simulink model "Sat_Nonliner_3"  (R2024a)
settings: Solver=ode45  StartTime=0.0  StopTime=20000  RelTol=1e-3  EnableMultiTasking=on
model workspace (MAT data in the model file):
  Q_fenzi = [2.841 -4.406 1.749]
values from neighbouring files (symbols this model uses):
  kzq_fenmu = kzq_fenmu_3    [Sat_Model_N_P.m]
  kzq_fenzi = kzq_fenzi_3    [Sat_Model_N_P.m]
  N_fenmu = N_fenmu_3    [Sat_Model_N_P.m]
  N_fenzi = N_fenzi_3    [Sat_Model_N_P.m]
  sat_alpha = sat_alpha_set_3_main(sat_alpha_i)    [SAT_MAIN.m]    (also in Sat_Model_G.m = 5; Sat_Model_N_P.m = sat_alpha_set(sat_alpha_i); model_sat_n_p.m = sat_alpha_1)
  T_fenmu = T_fenmu_3    [Sat_Model_N_P.m]
  T_fenzi = T_fenzi_3    [Sat_Model_N_P.m]
settings Model: Creator=75499  LastModifiedBy=xthinking
settings SolverCC: AlgebraicLoopSolver=TrustRegion
settings DataIOCC: LimitDataPoints=on  SaveFormat=Array  SignalLoggingSaveFormat=ModelDataLogs  ReturnWorkspaceOutputs=off
settings OptimizationCC: ExpressionDepthLimit=2147483647  LifeSpan=inf
settings DebuggingCC: UnderspecifiedInitializationDetection=Classic  MergeDetectMultiDrivingBlocksExec=none  SolverPrmCheckMsg=warning  FcnCallInpInsideContextMsg=warning  UnconnectedInputMsg=warning  UnconnectedOutputMsg=warning  UnconnectedLineMsg=warning  StateNameClashWarn=warning  SFUnexpectedBacktrackingDiag=warning  SFNoUnconditionalDefaultTransitionDiag=warning  SFExecutionAtInitializationDiag=none  ArithmeticOperatorsInVariantConditions=warning
settings HardwareCC: ProdBitPerPointer=32  ProdBitPerSizeT=32  ProdBitPerPtrDiffT=32  ProdLargestAtomicFloat=None  ProdIntDivRoundTo=Undefined  ProdEndianess=Unspecified  ProdWordSize=32  ProdHWDeviceType=32-bit Generic
settings ModelReferenceCC: EnableRefExpFcnMdlSchedulingChecks=on  PropagateSignalLabelsOutOfModel=off
settings SFSimCC: SimUseLocalCustomCode=off  CustomCodeUndefinedFunction=UseInterfaceOnly
settings RTWCC: RTWUseLocalCustomCode=off  GPUComputeCapability=3.5
settings CodeAppCC: StateflowObjectComments=on
settings GRTTargetCC: TargetLangStandard=C89/C90 (ANSI)
settings ConfigComp: CovMetricSettings=dw  CovSaveCumulativeToWorkspaceVar=on  CovSaveSingleToWorkspaceVar=on  CovExternalEMLEnable=off

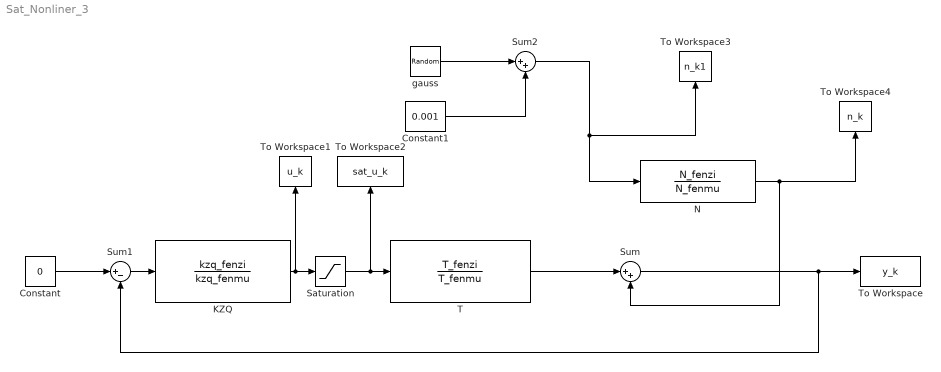
== system Sat_Nonliner_3 ==
  Constant : Constant  Value=0
  Constant1 : Constant  Value=0.001
  KZQ : DiscreteFilter  Numerator=kzq_fenzi  Denominator=kzq_fenmu
  N : DiscreteFilter  Numerator=N_fenzi  Denominator=N_fenmu
  Saturation : Saturate  UpperLimit=sat_alpha  LowerLimit=-sat_alpha  ZeroCross=off
  Sum : Sum  Inputs=|++
  Sum1 : Sum  Inputs=|+-
  Sum2 : Sum  Inputs=|++
  T : DiscreteFilter  Numerator=T_fenzi  Denominator=T_fenmu
  To Workspace : ToWorkspace  VariableName=y_k  SampleTime=-1
  To Workspace1 : ToWorkspace  VariableName=u_k  SampleTime=-1
  To Workspace2 : ToWorkspace  VariableName=sat_u_k  SampleTime=-1
  To Workspace3 : ToWorkspace  VariableName=n_k1  SampleTime=-1
  To Workspace4 : ToWorkspace  VariableName=n_k  SampleTime=-1
  gauss : RandomNumber  SampleTime=0.1
  wires:
  T/1 -> Sum/1
  N/1 -> Sum/2, To Workspace4/1
  Sum/1 -> To Workspace/1, Sum1/2
  Constant/1 -> Sum1/1
  Sum1/1 -> KZQ/1
  Saturation/1 -> T/1, To Workspace2/1
  KZQ/1 -> Saturation/1, To Workspace1/1
  gauss/1 -> Sum2/1
  Constant1/1 -> Sum2/2
  Sum2/1 -> To Workspace3/1, N/1
